simulink model "Main_model"  (R2021b)
settings: Solver=ode23t  StartTime=0.0  StopTime=sim_t_end  RelTol=1e-3
undefined symbols (not defined in the file): ambient_co2, ambient_pressure, ambient_rh, ambient_temp, battery, battery_heat_gen_scale, battery_mass, battery_thermal_mass, cab_air_v_dot, cabin_heater_cmd, cabin_heater_max_power, case_cold_plate_mass, case_cold_plate_thermal_mass, chiller_baffles_n, chiller_tube_length, chiller_tubes_n_rows, compressor_max_m_dot, compressor_ref_m_dot, condenser_air_min_flow_area, condenser_tube_width, const_current, coolant_channel_length, coolant_initial_T, coolant_m_dot, coolant_pipe_cross_sec_area, evaporator_air_cross_sec_area, evaporator_air_min_flow_area, evaporator_tube_width, motor_mc_heat_fraction, n_parallel, power_fraction_rear, ptc_heater_max_power, ptc_heater_thermal_mass, rad_air_v_dot, radiator_air_cross_sec_area, radiator_air_min_flow_area, radiator_tube_width, ref_m_dot, ref_pipe_dia, refrigerant_initial_void_fraction, refrigerant_pipe_cross_sec_area, T_bat_active_cool, T_bat_active_heat, T_bat_passive_cool, T_bat_passive_heat, T_battery_init, T_battery_nom, T_cabin_init, T_cabin_setpoint, T_dcdc_nom, T_DT_high, T_DT_passive_cool, T_DT_whr_active, T_front_gb_nom, T_front_mc_nom, T_front_motor_nom, T_rear_gb_nom, T_rear_mc_nom, T_rear_motor_nom, three_w_valve_max_open_area_factor ... (+3)
libraries: fl_lib x448, nesl_utility x328, SimscapeFluids_lib x134, slpidlib x15, ee_lib x9, simulink x8, LiBatteryElements_lib x4, SignalEditorBlockLib x1
(part 1 of 24)
settings Model: SimulationMode=accelerator  Creator=sagar  LastModifiedBy=sagar
settings SolverCC: MaxConsecutiveMinStep=3
settings DataIOCC: OutputOption=SpecifiedOutputTimes  OutputTimes=[0.25:0.25:sim_t_end-.25]
settings SimscapeCC: SimscapeLogType=all  SimscapeLogSimulationStatistics=on  SimscapeLogOpenViewer=on  SimscapeLogLimitData=off

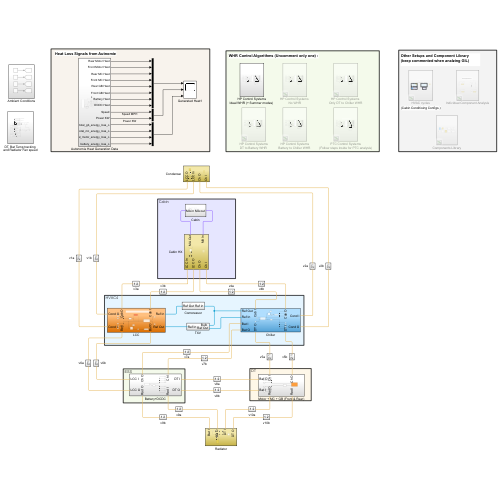
[thumbnail: Simulink's stored preview of the top-level diagram]
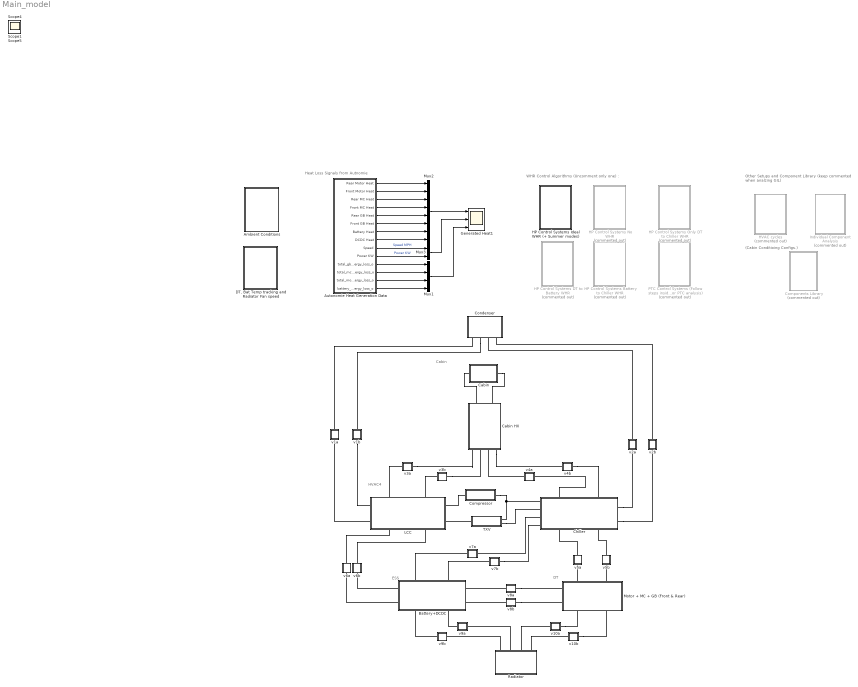
== system Main_model ==
  note: (Cabin Conditioing Configs.)
  note: WHR Control Algorithms (Uncomment only one) :
  note: ESS
  note: DT
  note: Cabin
  note: HVAC4
  note: Heat Loss Signals from Autnomie
  note: Other Setups and Component Library (keep commented when analzing GIL)
  Ambient Conditions : Subsystem
  Autonomie Heat Generation Data : Subsystem
  Battery+DCDC : Subsystem
      settings: PortSchema="{\"entries\":[{\"content\":{\"sides\":[{\"content\":{\"connectorIds\":[\"LConn1\",\"LConn2\"]},\"type\":\"ConnectorPlacement.EquallySpacedRectSide\",\"uuid\":\"0306e924-1f6f-4ced-9099-5caecc2870b0\"},{\"content\":{\"connectorIds\":[\"RConn1\",\"RConn2\"],\"side\":\"RIGHT\"},\"type\":\"ConnectorPlacement.EquallySpacedRectSide\",\"uuid\":\"35cdf91d-6fe2-4d3e-b00d-767662ac3c7b\"},{\"content\":{\"connectorIds\":[\"LConn3\",\"LConn4\"],\"side\":\"TOP\"},\"type\":\"ConnectorPlacement.EquallySpacedRectSide\",\"uuid\":\"83157bb8-78d9-4b65-8dba-e019d4108df5\"},{\"content\":{\"connectorIds\":[\"RConn3\",\"RConn4\"],\"side\":\"BOTTOM\"},\"type\":\"ConnectorPlacement.EquallySpacedRectSide\",\"uuid\":\"29cd2993-ed36-4139-acee-b229c5ae2169\"}]},\"type\":\"ConnectorPlacement.EquallySpacedConnector\",\"uuid\":\"a215272d-c7a6-45b8-87dc-b43228714672\"}],\"packageUris\":[\"http://schema.mathworks.com/mf0/Connector/R2020b\"],\"version\":\"1.0\"}"
  Cabin : Subsystem
  Cabin HX : Subsystem
  Chiller : Subsystem
      settings: PortSchema="{\"entries\":[{\"content\":{\"sides\":[{\"content\":{\"connectorIds\":[\"LConn1\",\"LConn2\"]},\"type\":\"ConnectorPlacement.EquallySpacedRectSide\",\"uuid\":\"a89dd059-1c83-4e1c-9fe3-39f2cb4f9afa\"},{\"content\":{\"connectorIds\":[\"RConn1\",\"RConn2\",\"RConn3\",\"RConn4\"],\"side\":\"RIGHT\"},\"type\":\"ConnectorPlacement.EquallySpacedRectSide\",\"uuid\":\"8c0c03c6-6d7a-4da4-915d-c6066f32c38c\"},{\"content\":{\"connectorIds\":[\"LConn3\",\"LConn4\"],\"side\":\"TOP\"},\"type\":\"ConnectorPlacement.EquallySpacedRectSide\",\"uuid\":\"f122d056-3fe7-4e3a-9529-4bff17fd05e4\"},{\"content\":{\"connectorIds\":[\"RConn5\",\"RConn6\"],\"side\":\"BOTTOM\"},\"type\":\"ConnectorPlacement.EquallySpacedRectSide\",\"uuid\":\"6a3b15ca-7f68-43b4-86bf-9ed13f068fa1\"}]},\"type\":\"ConnectorPlacement.EquallySpacedConnector\",\"uuid\":\"1dab3d5e-5f7c-4cee-857b-0b393e7503ec\"}],\"packageUris\":[\"http://schema.mathworks.com/mf0/Connector/R2020b\"],\"version\":\"1.0\"}"
  Components Library : Subsystem  Commented=on
  Compressor : Subsystem
  Condenser : Subsystem
  "DT, Bat Temp tracking and Radiator Fan speed" : Subsystem
  Generated Heat1 : Scope  NumInputPorts=3
  "HP Control Systems Battery to Chiller WHR " : Subsystem  Commented=on
  "HP Control Systems DT to Battery WHR " : Subsystem  Commented=on
  "HP Control Systems Ideal WHR (+ Summer modes) " : Subsystem
  HP Control Systems No WHR : Subsystem  Commented=on
  HP Control Systems Only DT to Chiller WHR : Subsystem  Commented=on
  HVAC cycles : Subsystem  Commented=on
  Individual Component Analysis : Subsystem  Commented=on
  LCC : Subsystem
      settings: PortSchema="{\"entries\":[{\"content\":{\"sides\":[{\"content\":{\"connectorIds\":[\"LConn1\",\"LConn2\"]},\"type\":\"ConnectorPlacement.EquallySpacedRectSide\",\"uuid\":\"c88537db-93e1-4260-954b-8033902de5a4\"},{\"content\":{\"connectorIds\":[\"RConn1\",\"RConn2\"],\"side\":\"RIGHT\"},\"type\":\"ConnectorPlacement.EquallySpacedRectSide\",\"uuid\":\"029d5487-6636-4cb7-8742-38b25d2e5ffc\"},{\"content\":{\"connectorIds\":[\"LConn3\",\"LConn4\"],\"side\":\"TOP\"},\"type\":\"ConnectorPlacement.EquallySpacedRectSide\",\"uuid\":\"ba351e7d-626c-49ed-814f-4dbb535f7b69\"},{\"content\":{\"connectorIds\":[\"RConn3\",\"RConn4\"],\"side\":\"BOTTOM\"},\"type\":\"ConnectorPlacement.EquallySpacedRectSide\",\"uuid\":\"04073c9d-6f46-40ac-b405-a599c04d4589\"}]},\"type\":\"ConnectorPlacement.EquallySpacedConnector\",\"uuid\":\"ae907a4e-6b91-45d2-b810-82f77aaed154\"}],\"packageUris\":[\"http://schema.mathworks.com/mf0/Connector/R2020b\"],\"version\":\"1.0\"}"
  Motor + MC + GB (Front & Rear) : Subsystem
      settings: PortSchema="{\"entries\":[{\"content\":{\"sides\":[{\"content\":{\"connectorIds\":[\"LConn1\",\"LConn2\"]},\"type\":\"ConnectorPlacement.EquallySpacedRectSide\",\"uuid\":\"c1d88535-5e48-4375-a89e-51b91784209e\"},{\"content\":{\"connectorIds\":[],\"side\":\"RIGHT\"},\"type\":\"ConnectorPlacement.EquallySpacedRectSide\",\"uuid\":\"9fddabb0-82e0-4708-8723-203cff57f397\"},{\"content\":{\"connectorIds\":[\"LConn3\",\"LConn4\"],\"side\":\"TOP\"},\"type\":\"ConnectorPlacement.EquallySpacedRectSide\",\"uuid\":\"c58e82b7-8199-4f57-9e5c-5b447251e46d\"},{\"content\":{\"connectorIds\":[\"RConn1\",\"RConn2\"],\"side\":\"BOTTOM\"},\"type\":\"ConnectorPlacement.EquallySpacedRectSide\",\"uuid\":\"9ef72b53-6421-43d8-9701-361e9df247e5\"}]},\"type\":\"ConnectorPlacement.EquallySpacedConnector\",\"uuid\":\"f9fcd3bb-8cab-462c-b7ba-6cef5d9b7fa5\"}],\"packageUris\":[\"http://schema.mathworks.com/mf0/Connector/R2020b\"],\"version\":\"1.0\"}"
  Mux1 : Mux
  Mux2 : Mux  Inputs=8
  Mux3 : Mux  Inputs=2
  PTC Control Systems (Follow steps inside for PTC analysis) : Subsystem  Commented=on
  Radiator : Subsystem
  TXV : Subsystem
  v10a : Subsystem
  v10b : Subsystem
  v1a : Subsystem
  v1b : Subsystem
  v2a : Subsystem
  v2b : Subsystem
  v3a : Subsystem
  v3b : Subsystem
  v4a : Subsystem
  v4b : Subsystem
  v5a : Subsystem
  v5b : Subsystem
  v6a : Subsystem
  v6b : Subsystem
  v7a : Subsystem
  v7b : Subsystem
  v8a : Subsystem
  v8b : Subsystem
  v9a : Subsystem
  v9b : Subsystem
  Scope1 : Scope
  Scope4 : Scope
  Scope5 : Scope
  wires:
  Mux3/1 -> Generated Heat1/2
  Mux2/1 -> Generated Heat1/1
  Autonomie Heat Generation Data/8(DCDC Heat) -> Mux2/8
  Autonomie Heat Generation Data/7(Battery Heat) -> Mux2/7
  Autonomie Heat Generation Data/6(Front GB Heat) -> Mux2/6
  Autonomie Heat Generation Data/5(Rear GB Heat) -> Mux2/5
  Autonomie Heat Generation Data/4(Front MC Heat) -> Mux2/4
  Autonomie Heat Generation Data/3(Rear MC Heat) -> Mux2/3
  Autonomie Heat Generation Data/2(Front Motor Heat) -> Mux2/2
  Autonomie Heat Generation Data/1(Rear Motor Heat) -> Mux2/1
  Autonomie Heat Generation Data/10(Power KW) -> Mux3/2  "Power KW"
  Autonomie Heat Generation Data/9(Speed) -> Mux3/1  "Speed MPH"
  Autonomie Heat Generation Data/11(total_gb_energy_loss_o) -> Mux1/1
  Autonomie Heat Generation Data/12(total_mc_energy_loss_o) -> Mux1/2
  Autonomie Heat Generation Data/13(total_motor_energy_loss_o) -> Mux1/3
  Autonomie Heat Generation Data/14(battery_energy_loss_o) -> Mux1/4
  Mux1/1 -> Generated Heat1/3
  connections:
  v6b/LConn1 -- LCC/RConn4
  LCC/LConn2 -- v1a/RConn1
  Radiator/RConn2 -- v9a/RConn1
  v10b/RConn1 -- Motor + MC + GB (Front & Rear)/RConn2
  v3a/RConn1 -- Cabin HX/RConn1
  Chiller/LConn2 -- v2b/RConn1
  v4b/RConn1 -- Chiller/LConn3
  v8a/LConn1 -- Battery+DCDC/RConn1
  v6a/LConn1 -- LCC/RConn3
  v7a/LConn1 -- Battery+DCDC/LConn3
  Motor + MC + GB (Front & Rear)/LConn3 -- v5a/RConn1
  v10a/RConn1 -- Motor + MC + GB (Front & Rear)/RConn1
  Chiller/RConn3 -- v7a/RConn1
  v1b/RConn1 -- LCC/LConn1
  Cabin/RConn1 -- Cabin HX/LConn1
  v5a/LConn1 -- Chiller/RConn6
  v2b/LConn1 -- Condenser/RConn4
  Chiller/LConn4 -- v4a/RConn1
  Chiller/LConn1 -- v2a/RConn1
  Radiator/RConn4 -- v10b/LConn1
  v5b/LConn1 -- Chiller/RConn5
  Radiator/RConn1 -- v9b/RConn1
  Cabin/LConn1 -- Cabin HX/LConn2
  Cabin HX/RConn4 -- v4b/LConn1
  LCC/LConn4 -- v3b/LConn1
  TXV/RConn1 -- LCC/RConn2
  LCC/LConn3 -- v3a/LConn1
  TXV/LConn2 -- Chiller/RConn2
  Condenser/RConn2 -- v1b/LConn1
  v8b/LConn1 -- Battery+DCDC/RConn2
  Battery+DCDC/LConn1 -- v6b/RConn1
  v4a/LConn1 -- Cabin HX/RConn3
  Battery+DCDC/LConn2 -- v6a/RConn1
  v3b/RConn1 -- Cabin HX/RConn2
  v8a/RConn1 -- Motor + MC + GB (Front & Rear)/LConn1
  Radiator/RConn3 -- v10a/LConn1
  Motor + MC + GB (Front & Rear)/LConn4 -- v5b/RConn1
  v9b/LConn1 -- Battery+DCDC/RConn3
  v7b/RConn1 -- Chiller/RConn4
  Battery+DCDC/LConn4 -- v7b/LConn1
  v9a/LConn1 -- Battery+DCDC/RConn4
  Chiller/RConn1 -- Compressor/RConn1 -- TXV/LConn1
  v8b/RConn1 -- Motor + MC + GB (Front & Rear)/LConn2
  Compressor/LConn1 -- LCC/RConn1
  v1a/LConn1 -- Condenser/RConn1
  v2a/LConn1 -- Condenser/RConn3

== system Main_model/Ambient Conditions ==
  CO2 Fraction : Constant  Value=ambient_co2
  Pressure : Constant  Value=ambient_pressure
  RH : Constant  Value=ambient_rh
  Temp : Constant  Value=ambient_temp
  tag scope: amb_P=global, amb_T=global, amb_co2=global, amb_rh=global
  wires:
  RH/1 -> [amb_rh]  "amb_rh"
  Pressure/1 -> [amb_P]  "amb_P"
  Temp/1 -> [amb_T]  "amb_T"
  CO2 Fraction/1 -> [amb_co2]  "amb_co2"

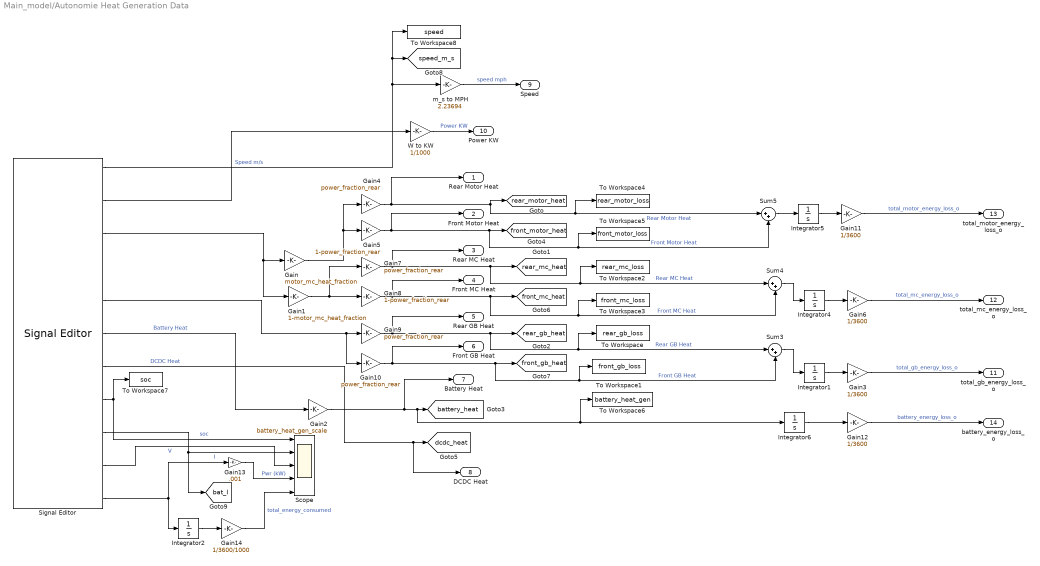
== system Main_model/Autonomie Heat Generation Data ==
  Gain : Gain  Gain=motor_mc_heat_fraction
  Gain1 : Gain  Gain=1-motor_mc_heat_fraction
  Gain{4,7,9..10} (4 alike) : Gain  Gain=power_fraction_rear
  Gain{3,6,11..12} (4 alike) : Gain  Gain=1/3600
  Gain13 : Gain  Gain=.001
  Gain14 : Gain  Gain=1/3600/1000
  Gain2 : Gain  Gain=battery_heat_gen_scale
  Gain5 : Gain  Gain=1-power_fraction_rear
  Gain8 : Gain  Gain=1-power_fraction_rear
  Integrator{1..2,4..6} (5 alike) : Integrator
  Scope : Scope  NumInputPorts=5
  Signal Editor : SignalEditorBlockLib/Signal Editor  FileName=C:\Users\sagar\OneDrive - University of Illinois - Urbana\Downloads\RA\Primary Ford Project\MATLAB Models\Model Ford Handover\Autonomie data processing\autonomie_drive_cycles_data.mat  ActiveScenario=us06_grade_0  ActiveSignal=speed  IsBus=off  OutputBusObjectStr=Bus: BusObject  SampleTime=0  Interpolate=off  ZeroCross=off  OutputAfterFinalValue=Setting to zero  Unit=inherit  PreserveSignalName=on
  Sum3 : Sum  Inputs=|++
  Sum4 : Sum  Inputs=|++
  Sum5 : Sum  Inputs=|++
  To Workspace : ToWorkspace  VariableName=rear_gb_loss  SaveFormat=Timeseries  SampleTime=-1
  To Workspace1 : ToWorkspace  VariableName=front_gb_loss  SaveFormat=Timeseries  SampleTime=-1
  To Workspace2 : ToWorkspace  VariableName=rear_mc_loss  SaveFormat=Timeseries  SampleTime=-1
  To Workspace3 : ToWorkspace  VariableName=front_mc_loss  SaveFormat=Timeseries  SampleTime=-1
  To Workspace4 : ToWorkspace  VariableName=rear_motor_loss  SaveFormat=Timeseries  SampleTime=-1
  To Workspace5 : ToWorkspace  VariableName=front_motor_loss  SaveFormat=Timeseries  SampleTime=-1
  To Workspace6 : ToWorkspace  VariableName=battery_heat_gen  SaveFormat=Timeseries  SampleTime=-1
  To Workspace7 : ToWorkspace  VariableName=soc  SaveFormat=Timeseries  SampleTime=-1
  To Workspace8 : ToWorkspace  VariableName=speed  SaveFormat=Timeseries  SampleTime=-1
  W to KW : Gain  Gain=1/1000
  m_s to MPH : Gain  Gain=2.23694
  Rear Motor Heat : Outport
  Front Motor Heat : Outport  Port=2
  Rear MC Heat : Outport  Port=3
  Front MC Heat : Outport  Port=4
  Rear GB Heat : Outport  Port=5
  Front GB Heat : Outport  Port=6
  Battery Heat : Outport  Port=7
  DCDC Heat : Outport  Port=8
  Speed : Outport  Port=9
  Power KW : Outport  Port=10
  total_gb_energy_loss_o : Outport  Port=11
  total_mc_energy_loss_o : Outport  Port=12
  total_motor_energy_loss_o : Outport  Port=13
  battery_energy_loss_o : Outport  Port=14
  tag scope: bat_I=global, battery_heat=global, dcdc_heat=global, front_gb_heat=global, front_mc_heat=global, front_motor_heat=global, rear_gb_heat=global, rear_mc_heat=global, rear_motor_heat=global, speed_m_s=global
  wires:
  Gain10/1 -> [front_gb_heat], To Workspace1/1, Sum3/2, Front GB Heat/1  "Front GB Heat"
  Signal Editor/5 -> Gain10/1, Gain9/1
  Gain9/1 -> To Workspace/1, Sum3/1, [rear_gb_heat], Rear GB Heat/1  "Rear GB Heat"
  Gain8/1 -> To Workspace3/1, Sum4/2, [front_mc_heat], Front MC Heat/1  "Front MC Heat"
  Gain7/1 -> To Workspace2/1, Sum4/1, [rear_mc_heat], Rear MC Heat/1  "Rear MC Heat"
  Signal Editor/7 -> [dcdc_heat], DCDC Heat/1  "DCDC Heat"
  Gain5/1 -> To Workspace5/1, Sum5/2, [front_motor_heat], Front Motor Heat/1  "Front Motor Heat"
  Signal Editor/6 -> Gain2/1  "Battery Heat"
  Signal Editor/3 -> Gain1/1, Gain/1
  Signal Editor/1 -> m_s to MPH/1, To Workspace8/1, [speed_m_s]  "Speed m/s"
  m_s to MPH/1 -> Speed/1  "speed mph"
  W to KW/1 -> Power KW/1  "Power KW"
  Signal Editor/2 -> W to KW/1
  Gain/1 -> Gain4/1, Gain5/1
  Gain1/1 -> Gain7/1, Gain8/1
  Gain2/1 -> To Workspace6/1, Integrator6/1, [battery_heat], Battery Heat/1
  Gain3/1 -> total_gb_energy_loss_o/1  "total_gb_energy_loss_o"
  Gain11/1 -> total_motor_energy_loss_o/1  "total_motor_energy_loss_o"
  Integrator5/1 -> Gain11/1
  Gain12/1 -> battery_energy_loss_o/1  "battery_energy_loss_o"
  Integrator6/1 -> Gain12/1
  Integrator1/1 -> Gain3/1
  Gain6/1 -> total_mc_energy_loss_o/1  "total_mc_energy_loss_o"
  Sum5/1 -> Integrator5/1
  Integrator4/1 -> Gain6/1
  Sum3/1 -> Integrator1/1
  Sum4/1 -> Integrator4/1
  Gain4/1 -> To Workspace4/1, Sum5/1, [rear_motor_heat], Rear Motor Heat/1  "Rear Motor Heat"
  Signal Editor/8 -> Scope/1, To Workspace7/1  "soc"
  Signal Editor/9 -> [bat_I], Scope/2  "I"
  Signal Editor/10 -> Scope/3  "V"
  Signal Editor/11 -> Integrator2/1, Gain13/1
  Gain13/1 -> Scope/4  "Pwr (kW)"
  Integrator2/1 -> Gain14/1
  Gain14/1 -> Scope/5  "total_energy_consumed"

== system Main_model/Battery+DCDC ==
  Battery+DCDC : Subsystem
  Pump : Subsystem
  LCC I : PMIOPort  Side=Left
  LCC O : PMIOPort  Port=2  Side=Left
  Ch O : PMIOPort  Port=3  Side=Left
  Ch I : PMIOPort  Port=4  Side=Left
  DT I : PMIOPort  Port=5  Side=Right
  DT O : PMIOPort  Port=6  Side=Right
  Rad O : PMIOPort  Port=7  Side=Right
  Rad I : PMIOPort  Port=8  Side=Right
  connections:
  Battery+DCDC/RConn1 -- Rad O/RConn1 -- DT O/RConn1 -- LCC O/RConn1 -- Ch O/RConn1
  Pump/RConn1 -- Battery+DCDC/RConn2
  Rad I/RConn1 -- DT I/RConn1 -- Pump/LConn1 -- LCC I/RConn1 -- Ch I/RConn1

== system Main_model/Cabin ==
  "\tconvection" : fl_lib/Thermal/Thermal Elements/Convective Heat Transfer  area=1 m^2  heat_tr_coeff=10 W/(m^2*K)  T_specify=off  T_priority=None  T=0 K  T_nominal_specify=off  T_nominal_unit=K  T_nominal_value=1  Q_specify=off  Q_priority=None  Q=0 W  Q_nominal_specify=off  Q_nominal_unit=W  Q_nominal_value=1
  Cabin Heat Transfer : Subsystem  Tag=PublishSubsystem  mask(Cabin Heat Transfer){glass_area=4, glass_thickness=0.004, glass_mass=3.5 * 0.004 * 2600, glass_specific_heat=840, glass_conductivity=0.96, glass_heat_coeff=40, glass_initial_temperature=T_cabin_init-273, doors_area=5, doors_thickness=0.06, doors_mass=75, doors_specific_heat=500, doors_conductivity=0.08, doors_heat_coeff=40, doors_initial_temperature=T_cabin_init-273, roof_area=3, roof_thickness=0.04, roof_mass=30, roof_specific_heat=500, roof_conductivity=0.08, roof_heat_coeff=40, roof_initial_temperature=T_cabin_init-273}
      mask prompts: glass_area "Area (m^2)"; glass_thickness "Thickness (m)"; glass_mass "Mass (kg)"; glass_specific_heat "Specific heat (J/kg/K)"; glass_conductivity "Thermal conductivity (W/m/K)"; glass_heat_coeff "Convective heat transfer coefficient (W/m^2/K)"; glass_initial_temperature "Initial temperature (degC)"; doors_area "Area (m^2)"; doors_thickness "Thickness (m)"; doors_mass "Mass (kg)"; doors_specific_heat "Specific heat (J/kg/K)"; doors_conductivity "Thermal conductivity (W/m/K)"; doors_heat_coeff "Convective heat transfer coefficient (W/m^2/K)"; doors_initial_temperature "Initial temperature (degC)"; roof_area "Area (m^2)"; roof_thickness "Thickness (m)"; roof_mass "Mass (kg)"; roof_specific_heat "Specific heat (J/kg/K)"; roof_conductivity "Thermal conductivity (W/m/K)"; roof_heat_coeff "Convective heat transfer coefficient (W/m^2/K)"; roof_initial_temperature "Initial temperature (degC)"
      mask DialogControl GlassTabVar Prompt: Glass
      mask DialogControl DoorsTabVar Prompt: Doors
      mask DialogControl RoofTabVar Prompt: Roof
  "Constant Volume Chamber (MA) " : fl_lib/Moist Air/Elements/Constant Volume Chamber (MA)  volume=4 m^3  num_ports=foundation.enum.num_ports.three  area_A=evaporator_air_cross_sec_area m^2  area_B=evaporator_air_cross_sec_area m^2  area_C=1.5 m^2  area_D=0.01 m^2  RH_ws=1  time_constant=1e-3 s  moisture_trace_gas_source=foundation.enum.moisture_trace_gas_source.none  moisture_source_spec=foundation.enum.moisture_source_spec.vapor  moisture_mass_flow=0 kg/s  moisture_temperature_spec=foundation.enum.temperature_spec.atmospheric  moisture_temperature=293.15 K  trace_gas_mass_flow=0 kg/s  trace_gas_temperature_spec=foundation.enum.temperature_spec.atmospheric  trace_gas_temperature=293.15 K  p_I_specify=on  p_I_priority=High  p_I=ambient_pressure MPa  p_I_nominal_specify=off  p_I_nominal_unit=MPa  p_I_nominal_value=1  T_I_specify=on  T_I_priority=High  T_I=T_cabin_init K  T_I_nominal_specify=off  T_I_nominal_unit=K  T_I_nominal_value=1  RH_I_specify=on  RH_I_priority=High  RH_I=ambient_rh  RH_I_nominal_specify=off  RH_I_nominal_unit=1  RH_I_nominal_value=1  x_w_I_specify=off  x_w_I_priority=None  x_w_I=0  x_w_I_nominal_specify=off  x_w_I_nominal_unit=1  x_w_I_nominal_value=1  y_w_I_specify=off  y_w_I_priority=None  y_w_I=0  y_w_I_nominal_specify=off  y_w_I_nominal_unit=1  y_w_I_nominal_value=1  HR_I_specify=off  HR_I_priority=None  HR_I=0  HR_I_nominal_specify=off  HR_I_nominal_unit=1  HR_I_nominal_value=1  x_g_I_specify=on  x_g_I_priority=None  x_g_I=0  x_g_I_nominal_specify=off  x_g_I_nominal_unit=1  x_g_I_nominal_value=1  y_g_I_specify=on  y_g_I_priority=High  y_g_I=ambient_co2  y_g_I_nominal_specify=off  y_g_I_nominal_unit=1  y_g_I_nominal_value=1
      settings: SourceProductBaseCode=SS  InternalSimscapePortConfiguration="{\"Bottom\":[],\"Left\":[{\"id\":\"A\",\"label\":\"A\",\"type\":\"foundation.moist_air.moist_air\"},{\"id\":\"B\",\"label\":\"B\",\"type\":\"foundation.moist_air.moist_air\"},{\"id\":\"C\",\"label\":\"C\",\"type\":\"foundation.moist_air.moist_air\"}],\"Right\":[{\"id\":\"W\",\"label\":\"W\",\"type\":\"output\"},{\"id\":\"F\",\"label\":\"F\",\"type\":\"output\"},{\"id\":\"H\",\"label\":\"H\",\"type\":\"foundation.thermal.thermal\"}],\"Top\":[]}"
  Controlled Heat Flow Rate Source : fl_lib/Thermal/Thermal Sources/Controlled Heat Flow Rate Source  Commented=on
  Controlled Reservoir (MA) : fl_lib/Moist Air/Elements/Controlled Reservoir (MA)  moisture_spec=foundation.enum.moisture_spec.relative_humidity  trace_gas_spec=foundation.enum.trace_gas_spec.mole_fraction  RH_ws=1  area_A=1.5 m^2  input_error_spec=foundation.enum.input_range_error.warn
      settings: SourceProductBaseCode=SS  InternalSimscapePortConfiguration="{\"Bottom\":[],\"Left\":[{\"id\":\"A\",\"label\":\"A\",\"type\":\"foundation.moist_air.moist_air\"}],\"Right\":[{\"id\":\"T\",\"label\":\"T\",\"type\":\"input\"},{\"id\":\"P\",\"label\":\"P\",\"type\":\"input\"},{\"id\":\"W\",\"label\":\"W\",\"type\":\"input\"},{\"id\":\"G\",\"label\":\"G\",\"type\":\"input\"}],\"Top\":[]}"
  Environment Temperature : fl_lib/Thermal/Thermal Sources/Controlled Temperature Source
  From6 : From  Commented=on  GotoTag=amb_T  TagVisibility=global
  From7 : From  Commented=on  GotoTag=T_cabin  TagVisibility=global
  Gain : Gain  Commented=on  Gain=100*1/30
  Gain1 : Gain  Commented=on  Gain=1/120
  Heat [W] : Gain  Gain=70
  Local Restriction (MA) : fl_lib/Moist Air/Elements/Local Restriction (MA)  restriction_type=foundation.enum.restriction_type.fixed  restriction_area=.005 m^2  min_area=1e-10 m^2  max_area=0.005 m^2  area=1.5 m^2  Cd=0.64  B_lam=0.999
      settings: SourceProductBaseCode=SS  InternalSimscapePortConfiguration="{\"Bottom\":[],\"Left\":[{\"id\":\"A\",\"label\":\"A\",\"type\":\"foundation.moist_air.moist_air\"}],\"Right\":[{\"id\":\"B\",\"label\":\"B\",\"type\":\"foundation.moist_air.moist_air\"}],\"Top\":[]}"
  Measurement Selector (MA) : fl_lib/Moist Air/Sensors/Measurement Selector (MA)  moisture_spec=foundation.enum.moisture_spec.relative_humidity  trace_gas_spec=foundation.enum.trace_gas_spec.mass_fraction
      settings: SourceProductBaseCode=SS
  Moist Air Properties (MA) : fl_lib/Moist Air/Utilities/Moist Air Properties (MA)  R_a=287.047 J/(K*kg)  T_TLU=[-56.55, -50 : 10 : -10, -5 : 1 : 5, 10 : 10 : 350]' degC  h_a_TLU=[342.416126230579; 349.005511058471; 359.063577249119; 369.119948684177; 379.175469465129; 389.230944678417; 394.258910928084; 395.264534937366; 396.27017101329; 397.275819932805; 398.281482472874; 399.287159410541; 400.292851523015; 401.298559587728; 402.304284382408; 403.310026685143; 404.315787274435; 409.34489180313; 419.404921755863; 429.468036401264; 439.535033154839; 449.606720928652; 459.683919949603; 469.767460521911; 479.858181001348; 489.956925196484; 500.064539372946; 510.181869006204; 520.309755403634; 530.449032296018; 540.60052248087; 550.765034584465; 560.943359995745; 571.136270013102; 581.344513234296; 591.568813210327; 601.809866375885; 612.068340261954; 622.344871990218; 632.640067043998; 642.95449830646; 653.288705353699; 663.643193987949; 674.018435994423; 684.414869104228; 694.832897145098; 705.272890361557; 715.735185886199; 726.220088344236; 736.727870574087; 747.258774447567; 757.813011774199] kJ/kg  mu_a_TLU=[14.2568883320012; 14.6140127728333; 15.1517277055779; 15.6806860159119; 16.2012351072083; 16.7137043125028; 16.9670071730589; 17.017438062815; 17.0677930842452; 17.1180725309876; 17.1682766951315; 17.2184058672268; 17.2684603362935; 17.3184403898301; 17.3683463138234; 17.4181783927569; 17.4679369096204; 17.7156358640698; 18.2056751785154; 18.68879035749; 19.1652344664982; 19.6352478927873; 20.099059103658; 20.5568853601578; 21.0089333871663; 21.4554000014051; 21.8964726992323; 22.3323302062775; 22.7631429910631; 23.1890737447833; 23.6102778293792; 24.0269036959922; 24.4390932757886; 24.8469823450548; 25.2507008663546; 25.6503733074314; 26.0461189394339; 26.4380521159325; 26.8262825340948; 27.2109154792923; 27.5920520543128; 27.969789394274; 28.3442208682439; 28.7154362685068; 29.0835219883356; 29.4485611890712; 29.8106339572472; 30.1698174524429; 30.5261860464955; 30.8798114546565; 31.2307628592324; 31.5791070262086] s*uPa  k_a_TLU=[19.8808489374933; 20.4162454629695; 21.2248743590758; 22.0232452890903; 22.8117314495857; 23.5906913619588; 23.9767075412237; 24.053639990175; 24.1304826682191; 24.2072359051629; 24.2839000294007; 24.3604753679152; 24.4369622462801; 24.5133609886625; 24.5896719178249; 24.6658953551279; 24.7420316205333; 25.1214164701832; 25.8738283029331; 26.6180150229276; 27.3542674377332; 28.0828634735341; 28.8040686837224; 29.5181367785657; 30.2253101618423; 30.9258204644224; 31.6198890677835; 32.3077276126633; 32.9895384896798; 33.6655153099498; 34.33584335461; 35.0007000027879; 35.6602551380254; 36.3146715334901; 36.9641052165342; 37.6087058133173; 38.248616874307; 38.8839761815308; 39.5149160384798; 40.1415635435708; 40.7640408480637; 41.3824653993118; 41.9969501701893; 42.6076038755117; 43.2145311762238; 43.8178328720941; 44.4176060836121; 45.013944423749; 45.6069381602018; 46.1966743687041; 46.783237077953; 47.3667074066625] mW/(K*m)  p_min=1 kPa  p_max=inf MPa  T_min=-56.55 degC  T_max=350 degC  p_atm=ambient_pressure MPa  T_atm=ambient_temp degC  R_w=461.523 J/(K*kg)  p_ws_TLU=[1.71168953425982e-06; 3.93770601979424e-06; 1.28411717710344e-05; 3.80051394873809e-05; .00010323902900209; .000259873810798063; .000401741022116384; .000437454836117844; .000476040820618202; .000517704666185737; .000562664883741207; .000611212677444345; .000657088049117899; .000705987905898279; .000758082381149132; .000813549384183233; .000872574861129522; .00122818386934022; .0023392147667769; .00424668834054807; .00738442748706953; .0123512704340234; .0199458019246787; .0312006356960619; .0474147199263783; .0701823607447713; .10141797792131; .143375967241115; .198665399739302; .270259606559999; .361500961984849; .476101381081492; .618139196722055; .792053183687694; 1.0026345688121; 1.25501792086105; 1.55467186826983; 1.90739066433297; 2.31928772772542; 2.79679245576864; 3.34665187151016; 3.97593907083533; 4.69207105435535; 5.5028394740883; 6.41645928168037; 7.4416425436169; 8.58770832955728; 9.86474556030261; 11.2838558865497; 12.8575218898034; 14.6001810568052; 16.5291642526045] MPa  h_w_vap_TLU=[2836.88241275372; 2837.81392500514; 2838.63937175807; 2838.7309929628; 2838.06905313927; 2836.62597341095; 2835.60023952573; 2835.37006381376; 2835.13143158077; 2834.88429145066; 2834.62859062897; 2500.93420564316; 2498.55329907119; 2496.17495082036; 2493.79885912205; 2491.42474723191; 2489.05236104642; 2477.20875029194; 2453.54955988604; 2429.83856603313; 2406.00136954922; 2381.97406342174; 2357.69101156389; 2333.08088387814; 2308.06565480412; 2282.56034405021; 2256.47287422313; 2229.70428017508; 2202.14968030993; 2173.69998896199; 2144.24368406447; 2113.66758247452; 2081.85585110571; 2048.68725710494; 2014.03141249899; 1977.7449923284; 1939.66849592886; 1899.62342931686; 1857.40930169838; 1812.79975416601; 1765.53721731251; 1715.32525772152; 1661.81700477787; 1604.59703745016; 1543.1534616334; 1476.83692476464; 1404.80240352424; 1325.92091736114; 1238.61667822208; 1140.5102987018; 1027.62017777647; 892.733785613825] kJ/kg  h_w_TLU=[2396.55944251649; 2408.68643343608; 2427.1988031141; 2445.702165897; 2464.18429108356; 2482.62529466839; 2491.82135326629; 2493.6580151792; 2495.49372578218; 2497.32843835745; 2499.16210446923; 2500.99462758899; 2502.83092214066; 2504.6665223621; 2506.50140563013; 2508.335548891; 2510.16892865793; 2519.32352241995; 2537.56068088674; 2555.67742615292; 2573.6403223998; 2591.4109179101; 2608.9455037701; 2626.19492016262; 2643.10444358428; 2659.61377634497; 2675.58278696023; 2696.1846256545; 2716.49989553741; 2736.6235210957; 2756.61216047011; 2776.50561773853; 2796.33378922508; 2816.11979583049; 2835.88181423877; 2855.63430574511; 2875.38889327595; 2895.15500577172; 2914.94035964689; 2934.75132290228; 2954.59319330244; 2974.47041285505; 2994.38673458964; 3014.34535328009; 3034.34900867103; 3054.40006755764; 3074.50058946898; 3094.65237953784; 3114.85703128106; 3135.11596137801; 3155.43043805905; 3175.80160435813] kJ/kg  mu_w_TLU=[6.81365662228272; 7.04953750742707; 7.40970098298307; 7.76991278093907; 8.13017290129507; 8.49048134405107; 8.67065368632907; 8.70668960445667; 8.74272600580827; 8.77876289038387; 8.81480025818347; 8.85083810920707; 8.88687644345467; 8.92291526092627; 8.95895456162187; 8.99499434554147; 9.03103461268507; 9.21124319676307; 9.57169660671907; 9.93219833907507; 10.2927483938311; 10.6533467709871; 11.0139934705431; 11.3746884924991; 11.7354318368551; 12.0962235036111; 12.4570634927671; 12.8179518043231; 13.1788884382791; 13.5398733946351; 13.9009066733911; 14.2619882745471; 14.6231181981031; 14.9842964440591; 15.3455230124151; 15.7067979031711; 16.0681211163271; 16.4294926518831; 16.7909125098391; 17.1523806901951; 17.5138971929511; 17.8754620181071; 18.2370751656631; 18.5987366356191; 18.9604464279751; 19.3222045427311; 19.6840109798871; 20.0458657394431; 20.4077688213991; 20.7697202257551; 21.1317199525111; 21.4937680016671] s*uPa  k_w_TLU=[11.46288215976; 11.941997488935; 12.676358586935; 13.414208884935; 14.155548382935; 14.900377080935; 15.274099879935; 15.348949115735; 15.423833243535; 15.498752263335; 15.573706175135; 15.648694978935; 15.723718674735; 15.798777262535; 15.873870742335; 15.948999114135; 16.024162377935; 16.400502076935; 17.155798374935; 17.914583872935; 18.676858570935; 19.442622468935; 20.211875566935; 20.984617864935; 21.760849362935; 22.540570060935; 23.323779958935; 24.110479056935; 24.900667354935; 25.694344852935; 26.491511550935; 27.292167448935; 28.096312546935; 28.903946844935; 29.715070342935; 30.529683040935; 31.347784938935; 32.169376036935; 32.994456334935; 33.823025832935; 34.655084530935; 35.490632428935; 36.329669526935; 37.172195824935; 38.018211322935; 38.867716020935; 39.720709918935; 40.577193016935; 41.437165314935; 42.300626812935; 43.167577510935; 44.038017408935] mW/(K*m)  D_w=25 mm^2/s  trace_gas_model=foundation.enum.trace_gas_model.none  R_g=188.923 J/(K*kg)  h_g_TLU=[439.555216260064; 444.670268200251; 452.538618847003; 460.487124258496; 468.522588768941; 476.649415958793; 480.74798538725; 481.57054318762; 482.394052398751; 483.218514288831; 484.043930029015; 484.870300696555; 485.697627277859; 486.525910671489; 487.355151691079; 488.185351068185; 489.016509455051; 493.186704139431; 501.599194953048; 510.107689961685; 518.711611080182; 527.410026793075; 536.201764778798; 545.085474203452; 554.059675505208; 563.122805485367; 572.27325096919; 581.509373027928; 590.829525105886; 600.232066705818; 609.715373581392; 619.277845178105; 628.917909922924; 638.634028838794; 648.424697859328; 658.288449140109; 668.223851601449; 678.229510889093; 688.304068901113; 698.44620299875; 708.654624994591; 718.928079991818; 729.265345132425; 739.665228299475; 750.126566808087; 760.648226111439; 771.229098541268; 781.868102096908; 792.564179292476; 803.316296068366; 814.123440770426; 824.984623198037] kJ/kg  mu_g_TLU=[10.8921054191698; 11.2215357085649; 11.7233300740382; 12.2234238147811; 12.7215124453467; 13.2173328890673; 13.4643203184773; 13.5136406274989; 13.562934752385; 13.6122025024997; 13.6614436900741; 13.7106581301692; 13.7598456406398; 13.8090060420983; 13.8581391578796; 13.9072448140062; 13.9563228391538; 14.2012926853717; 14.6890687376044; 15.1738428124161; 15.6554929043332; 16.1339159800463; 16.6090257998657; 17.0807510097148; 17.5490334645512; 18.0138267508952; 18.4750948814453; 18.9328111390399; 19.3869570507278; 19.8375214755778; 20.2844997922255; 20.7278931741254; 21.1677079421287; 21.6039549853963; 22.036649242835; 22.4658092382469; 22.8914566632375; 23.3136160026627; 23.7323141980278; 24.1475803447965; 24.5594454200432; 24.9679420372927; 25.3731042257492; 25.774967231431; 26.1735673380029; 26.5689417053362; 26.9611282240413; 27.350165384404; 27.73609215832; 28.118947892972; 28.4987722151178; 28.8756049449796] s*uPa  k_g_TLU=[10.489430678843; 10.9507672150864; 11.666197960308; 12.392559739764; 13.1299519771612; 13.8778409888416; 14.2554325416312; 14.3312274189707; 14.4071122346908; 14.4830860227061; 14.5591478179508; 14.6352966574703; 14.7115315815553; 14.787851634907; 14.8642558678259; 14.9407433374142; 15.0173131087819; 15.401364480906; 16.1751373988038; 16.9558134611595; 17.7432208682398; 18.5366976599676; 19.3360988502003; 20.1412225692689; 20.9517507672929; 21.7672310558863; 22.5871115634685; 23.4107980865695; 24.2377021890869; 25.0672663781241; 25.8989689893876; 26.732318357514; 27.5668446164644; 28.4020933015927; 29.2376215872816; 30.0729965057542; 30.9077942826816; 31.7416001931033; 32.5740086297993; 33.4046232539953; 34.2330571812868; 35.0589331874899; 35.8818839295189; 36.701552179391; 37.5175910702657; 38.3296643536716; 39.1374466671854; 39.9406238119064; 40.7388930391313; 41.5319633456945; 42.3195557774861; 43.1014037407076] mW/(K*m)  D_g=16 mm^2/s
      settings: SourceProductBaseCode=SS
  N_passengers : Constant  Value=2
  Occupant Heat Gain : fl_lib/Thermal/Thermal Sources/Controlled Heat Flow Rate Source
  PS-Simulink Converter : nesl_utility/PS-Simulink Converter  PhysicalDomain=network_engine_domain  SubClassName=ps_output  LeftPortType=input  RightPortType=output  PseudoPeriodic=off  Frequencies=[]  Unit=inherit  AffineConversion=off
      settings: SourceProductBaseCode=PW,SS
  PS-Simulink Converter1 : nesl_utility/PS-Simulink Converter  PhysicalDomain=network_engine_domain  SubClassName=ps_output  LeftPortType=input  RightPortType=output  PseudoPeriodic=off  Frequencies=[]  Unit=inherit  AffineConversion=off
      settings: SourceProductBaseCode=PW,SS
  Ramp : simulink/Sources/Ramp  Commented=on  slope=-20/10000  start=0  InitialOutput=-1
  Seat and other Convection : fl_lib/Thermal/Thermal Elements/Convective Heat Transfer  area=5 m^2  heat_tr_coeff=60 W/(m^2*K)  T_specify=off  T_priority=None  T=0 K  T_nominal_specify=off  T_nominal_unit=K  T_nominal_value=1  Q_specify=off  Q_priority=None  Q=0 W  Q_nominal_specify=off  Q_nominal_unit=W  Q_nominal_value=1
  Simulink-PS Converter : nesl_utility/Simulink-PS Converter  PhysicalDomain=network_engine_domain  SubClassName=ps_input  LeftPortType=input  RightPortType=output  PseudoPeriodic=off  Frequencies=[]  NoiseDistribution=none  NoiseParameters=[]  Unit=K  AffineConversion=off  FilteringAndDerivatives=provide  SimscapeFilterOrder=1  InputFilterTimeConstant=0.001  UdotUserProvided=0
      settings: SourceProductBaseCode=PW,SS
  Simulink-PS Converter1 : nesl_utility/Simulink-PS Converter  PhysicalDomain=network_engine_domain  SubClassName=ps_input  LeftPortType=input  RightPortType=output  PseudoPeriodic=off  Frequencies=[]  NoiseDistribution=none  NoiseParameters=[]  Unit=MPa  AffineConversion=off  FilteringAndDerivatives=provide  SimscapeFilterOrder=1  InputFilterTimeConstant=0.001  UdotUserProvided=0
      settings: SourceProductBaseCode=PW,SS
  Simulink-PS Converter2 : nesl_utility/Simulink-PS Converter  PhysicalDomain=network_engine_domain  SubClassName=ps_input  LeftPortType=input  RightPortType=output  PseudoPeriodic=off  Frequencies=[]  NoiseDistribution=none  NoiseParameters=[]  Unit=1  AffineConversion=off  FilteringAndDerivatives=provide  SimscapeFilterOrder=1  InputFilterTimeConstant=0.001  UdotUserProvided=0
      settings: SourceProductBaseCode=PW,SS
  Simulink-PS Converter3 : nesl_utility/Simulink-PS Converter  PhysicalDomain=network_engine_domain  SubClassName=ps_input  LeftPortType=input  RightPortType=output  PseudoPeriodic=off  Frequencies=[]  NoiseDistribution=none  NoiseParameters=[]  Unit=1  AffineConversion=off  FilteringAndDerivatives=provide  SimscapeFilterOrder=1  InputFilterTimeConstant=0.001  UdotUserProvided=0
      settings: SourceProductBaseCode=PW,SS
  Simulink-PS Converter4 : nesl_utility/Simulink-PS Converter  Commented=on  PhysicalDomain=network_engine_domain  SubClassName=ps_input  LeftPortType=input  RightPortType=output  PseudoPeriodic=off  Frequencies=[]  NoiseDistribution=none  NoiseParameters=[]  Unit=kW  AffineConversion=off  FilteringAndDerivatives=provide  SimscapeFilterOrder=1  InputFilterTimeConstant=0.001  UdotUserProvided=0
      settings: SourceProductBaseCode=PW,SS
  Simulink-PS Converter5 : nesl_utility/Simulink-PS Converter  PhysicalDomain=network_engine_domain  SubClassName=ps_input  LeftPortType=input  RightPortType=output  PseudoPeriodic=off  Frequencies=[]  NoiseDistribution=none  NoiseParameters=[]  Unit=K  AffineConversion=on  FilteringAndDerivatives=provide  SimscapeFilterOrder=1  InputFilterTimeConstant=0.001  UdotUserProvided=0
      settings: SourceProductBaseCode=PW,SS
  Simulink-PS Converter8 : nesl_utility/Simulink-PS Converter  PhysicalDomain=network_engine_domain  SubClassName=ps_input  LeftPortType=input  RightPortType=output  PseudoPeriodic=off  Frequencies=[]  NoiseDistribution=none  NoiseParameters=[]  Unit=W  AffineConversion=off  FilteringAndDerivatives=provide  SimscapeFilterOrder=1  InputFilterTimeConstant=0.001  UdotUserProvided=0
      settings: SourceProductBaseCode=PW,SS
  Subtract : Sum  Commented=on  Inputs=+-
  Switch1 : Switch  Commented=on  Criteria=u2 > Threshold
  Temperature Sensor : fl_lib/Thermal/Thermal Sensors/Temperature Sensor
  Thermal Mass : fl_lib/Thermal/Thermal Elements/Thermal Mass  mass=150 kg  sp_heat=600 J/(K*kg)  T_specify=on  T_priority=High  T=T_cabin_init K  T_nominal_specify=off  T_nominal_unit=K  T_nominal_value=1  Q_specify=off  Q_priority=None  Q=0 W  Q_nominal_specify=off  Q_nominal_unit=W  Q_nominal_value=1
  Thermal Mass1 : fl_lib/Thermal/Thermal Elements/Thermal Mass  mass=2 kg  sp_heat=600 J/(K*kg)  T_specify=on  T_priority=High  T=T_cabin_init K  T_nominal_specify=off  T_nominal_unit=K  T_nominal_value=1  Q_specify=off  Q_priority=None  Q=0 W  Q_nominal_specify=off  Q_nominal_unit=W  Q_nominal_value=1
  Thermal Reference : fl_lib/Thermal/Thermal Elements/Thermal Reference  Commented=on
  Thermal Reference1 : fl_lib/Thermal/Thermal Elements/Thermal Reference
  Thermal Reference2 : fl_lib/Thermal/Thermal Elements/Thermal Reference
  Thermal Reference3 : fl_lib/Thermal/Thermal Elements/Thermal Reference
  To Workspace : ToWorkspace  VariableName=T_cabin  SaveFormat=Timeseries  SampleTime=-1
  Transfer Fcn1 : TransferFcn  Commented=on  Denominator=[1 1]
  MA out : PMIOPort  Side=Left
  MA in : PMIOPort  Port=2  Side=Right
  tag scope: T_cabin=global
  wires:
  Ramp/1 -> Simulink-PS Converter4/1
  N_passengers/1 -> Heat [W]/1
  Heat [W]/1 -> Simulink-PS Converter8/1
  [amb_T] -> Simulink-PS Converter5/1
  Gain1/1 -> Switch1/3
  Gain/1 -> Switch1/1
  Switch1/1 -> Transfer Fcn1/1
  Subtract/1 -> Switch1/2, Gain/1, Gain1/1
  From7/1 -> Subtract/2
  From6/1 -> Subtract/1
  PS-Simulink Converter/1 -> [T_cabin]
  [amb_P] -> Simulink-PS Converter1/1
  [amb_co2] -> Simulink-PS Converter3/1
  [amb_rh] -> Simulink-PS Converter2/1
  [amb_T] -> Simulink-PS Converter/1
  PS-Simulink Converter1/1 -> To Workspace/1
  connections:
  Environment Temperature/LConn1 -- Cabin Heat Transfer/RConn1
  Simulink-PS Converter8/RConn1 -- Occupant Heat Gain/RConn1
  Simulink-PS Converter5/RConn1 -- Environment Temperature/RConn1
  Thermal Reference1/LConn1 -- Occupant Heat Gain/RConn2
  Thermal Reference2/LConn1 -- Environment Temperature/RConn2
  Cabin Heat Transfer/LConn1 -- "\tconvection"/RConn1 -- "Constant Volume Chamber (MA) "/RConn3 -- Controlled Heat Flow Rate Source/LConn1 -- Seat and other Convection/RConn1 -- Occupant Heat Gain/LConn1
  Controlled Heat Flow Rate Source/RConn1 -- Simulink-PS Converter4/RConn1
  PS-Simulink Converter/LConn1 -- Measurement Selector (MA)/RConn2
  "Constant Volume Chamber (MA) "/RConn2 -- Measurement Selector (MA)/LConn1
  Thermal Reference/LConn1 -- Controlled Heat Flow Rate Source/RConn2
  MA out/RConn1 -- "Constant Volume Chamber (MA) "/LConn2
  MA in/RConn1 -- "Constant Volume Chamber (MA) "/LConn1
  Thermal Mass/LConn1 -- Seat and other Convection/LConn1
  Local Restriction (MA)/LConn1 -- Moist Air Properties (MA)/RConn1 -- Controlled Reservoir (MA)/LConn1
  Simulink-PS Converter2/RConn1 -- Controlled Reservoir (MA)/RConn3
  Simulink-PS Converter3/RConn1 -- Controlled Reservoir (MA)/RConn4
  Simulink-PS Converter1/RConn1 -- Controlled Reservoir (MA)/RConn2
  Simulink-PS Converter/RConn1 -- Controlled Reservoir (MA)/RConn1
  Local Restriction (MA)/RConn1 -- "Constant Volume Chamber (MA) "/LConn3
  Thermal Mass1/LConn1 -- "\tconvection"/LConn1 -- Temperature Sensor/LConn1
  Temperature Sensor/RConn1 -- Thermal Reference3/LConn1
  PS-Simulink Converter1/LConn1 -- Temperature Sensor/RConn2

== system Main_model/Cabin HX ==
  Pump : Subsystem
  cabin_hx : Subsystem
      settings: PortSchema="{\"entries\":[{\"content\":{\"sides\":[{\"content\":{\"connectorIds\":[]},\"type\":\"ConnectorPlacement.EquallySpacedRectSide\",\"uuid\":\"71822b2c-9ca3-4cc9-92d1-ecf472f04bd4\"},{\"content\":{\"connectorIds\":[],\"side\":\"RIGHT\"},\"type\":\"ConnectorPlacement.EquallySpacedRectSide\",\"uuid\":\"e0df667d-86dd-460a-bd26-f563eb1ee1db\"},{\"content\":{\"connectorIds\":[\"LConn1\",\"LConn2\"],\"side\":\"TOP\"},\"type\":\"ConnectorPlacement.EquallySpacedRectSide\",\"uuid\":\"56daad42-8202-443d-af27-a6baa0bd3366\"},{\"content\":{\"connectorIds\":[\"RConn1\",\"RConn2\"],\"side\":\"BOTTOM\"},\"type\":\"ConnectorPlacement.EquallySpacedRectSide\",\"uuid\":\"4778d153-f81a-4fb0-9678-a5e1ef62924d\"}]},\"type\":\"ConnectorPlacement.EquallySpacedConnector\",\"uuid\":\"488efe04-0e39-4e1b-8b30-4bca48b36ba3\"}],\"packageUris\":[\"http://schema.mathworks.com/mf0/Connector/R2020b\"],\"version\":\"1.0\"}"
  cabin_hx1 : Subsystem  Commented=on
      settings: PortSchema="{\"entries\":[{\"content\":{\"sides\":[{\"content\":{\"connectorIds\":[]},\"type\":\"ConnectorPlacement.EquallySpacedRectSide\",\"uuid\":\"71822b2c-9ca3-4cc9-92d1-ecf472f04bd4\"},{\"content\":{\"connectorIds\":[],\"side\":\"RIGHT\"},\"type\":\"ConnectorPlacement.EquallySpacedRectSide\",\"uuid\":\"e0df667d-86dd-460a-bd26-f563eb1ee1db\"},{\"content\":{\"connectorIds\":[\"LConn1\",\"LConn2\"],\"side\":\"TOP\"},\"type\":\"ConnectorPlacement.EquallySpacedRectSide\",\"uuid\":\"56daad42-8202-443d-af27-a6baa0bd3366\"},{\"content\":{\"connectorIds\":[\"RConn1\",\"RConn2\"],\"side\":\"BOTTOM\"},\"type\":\"ConnectorPlacement.EquallySpacedRectSide\",\"uuid\":\"4778d153-f81a-4fb0-9678-a5e1ef62924d\"}]},\"type\":\"ConnectorPlacement.EquallySpacedConnector\",\"uuid\":\"488efe04-0e39-4e1b-8b30-4bca48b36ba3\"}],\"packageUris\":[\"http://schema.mathworks.com/mf0/Connector/R2020b\"],\"version\":\"1.0\"}"
  MA Out : PMIOPort  Side=Left
  MA In : PMIOPort  Port=2  Side=Left
  LCC In : PMIOPort  Port=3  Side=Right
  LCC O : PMIOPort  Port=4  Side=Right
  Ch O : PMIOPort  Port=5  Side=Right
  Ch I : PMIOPort  Port=6  Side=Right
  connections:
  cabin_hx/LConn1 -- MA In/RConn1
  LCC In/RConn1 -- Pump/LConn1 -- Ch I/RConn1
  cabin_hx/LConn2 -- MA Out/RConn1
  LCC O/RConn1 -- cabin_hx/RConn2 -- Ch O/RConn1
  cabin_hx/RConn1 -- Pump/RConn1

== system Main_model/Chiller ==
  Absolute Reference (TL) : fl_lib/Thermal Liquid/Elements/Absolute Reference (TL)
      settings: SourceProductBaseCode=SS
  PS-Simulink Converter : nesl_utility/PS-Simulink Converter  PhysicalDomain=network_engine_domain  SubClassName=ps_output  LeftPortType=input  RightPortType=output  PseudoPeriodic=off  Frequencies=[]  Unit=inherit  AffineConversion=off
      settings: SourceProductBaseCode=PW,SS
  Pressure & Temperature Sensor (TL) : fl_lib/Thermal Liquid/Sensors/Pressure & Temperature Sensor (TL)
      settings: SourceProductBaseCode=SS  InternalSimscapePortConfiguration="{\"Bottom\":[],\"Left\":[{\"id\":\"A\",\"label\":\"A\",\"type\":\"foundation.thermal_liquid.thermal_liquid\"}],\"Right\":[{\"id\":\"B\",\"label\":\"B\",\"type\":\"foundation.thermal_liquid.thermal_liquid\"},{\"id\":\"P\",\"label\":\"P\",\"type\":\"output\"},{\"id\":\"T\",\"label\":\"T\",\"type\":\"output\"}],\"Top\":[]}"
  Pump : Subsystem
  chiller : Subsystem
  Cond I : PMIOPort  Side=Left
  Cond O : PMIOPort  Port=2  Side=Left
  Cab O : PMIOPort  Port=3  Side=Left
  Cab I : PMIOPort  Port=4  Side=Left
  Ref Out : PMIOPort  Port=5  Side=Right
  Ref In : PMIOPort  Port=6  Side=Right
  Bat I : PMIOPort  Port=7  Side=Right
  Bat O : PMIOPort  Port=8  Side=Right
  DT I : PMIOPort  Port=9  Side=Right
  DT O : PMIOPort  Port=10  Side=Right
  tag scope: T_chiller_out=global
  wires:
  PS-Simulink Converter/1 -> [T_chiller_out]
  connections:
  Pump/RConn1 -- chiller/LConn2
  chiller/LConn1 -- Pressure & Temperature Sensor (TL)/LConn1 -- DT O/RConn1 -- Bat O/RConn1 -- Cond O/RConn1 -- Cab O/RConn1
  chiller/RConn1 -- Ref Out/RConn1
  Ref In/RConn1 -- chiller/RConn2
  DT I/RConn1 -- Pump/LConn1 -- Cond I/RConn1 -- Cab I/RConn1 -- Bat I/RConn1
  Absolute Reference (TL)/LConn1 -- Pressure & Temperature Sensor (TL)/RConn1
  PS-Simulink Converter/LConn1 -- Pressure & Temperature Sensor (TL)/RConn3

== system Main_model/Components Library ==
  4-w valve : Subsystem  Commented=on
  Compressor : Subsystem  Commented=on
  LCC : Subsystem  Commented=on
  Miscellaneous Components : Subsystem  Commented=on
  TXV : Subsystem  Commented=on
  cabin : Subsystem  Commented=on
  cabin HX : Subsystem  Commented=on
      settings: PortSchema="{\"entries\":[{\"content\":{\"sides\":[{\"content\":{\"connectorIds\":[]},\"type\":\"ConnectorPlacement.EquallySpacedRectSide\",\"uuid\":\"71822b2c-9ca3-4cc9-92d1-ecf472f04bd4\"},{\"content\":{\"connectorIds\":[],\"side\":\"RIGHT\"},\"type\":\"ConnectorPlacement.EquallySpacedRectSide\",\"uuid\":\"e0df667d-86dd-460a-bd26-f563eb1ee1db\"},{\"content\":{\"connectorIds\":[\"LConn1\",\"LConn2\"],\"side\":\"TOP\"},\"type\":\"ConnectorPlacement.EquallySpacedRectSide\",\"uuid\":\"56daad42-8202-443d-af27-a6baa0bd3366\"},{\"content\":{\"connectorIds\":[\"RConn1\",\"RConn2\"],\"side\":\"BOTTOM\"},\"type\":\"ConnectorPlacement.EquallySpacedRectSide\",\"uuid\":\"4778d153-f81a-4fb0-9678-a5e1ef62924d\"}]},\"type\":\"ConnectorPlacement.EquallySpacedConnector\",\"uuid\":\"488efe04-0e39-4e1b-8b30-4bca48b36ba3\"}],\"packageUris\":[\"http://schema.mathworks.com/mf0/Connector/R2020b\"],\"version\":\"1.0\"}"
  cabin evap : Subsystem  Commented=on
  chiller : Subsystem  Commented=on
  condenser : Subsystem  Commented=on
  pump : Subsystem  Commented=on
  radiator : Subsystem  Commented=on
